simulink model "adrc_plant"  (R2026a)
settings: Solver=FixedStepDiscrete  StartTime=0  StopTime=6  FixedStep=0.004
settings Model: Creator=Aethor_ca  LastModifiedBy=Aethor_ca
settings DebuggingCC: AlgebraicLoopMsg=error
settings ModelReferenceCC: ModelReferenceMinAlgLoopOccurrences=on
settings GRTTargetCC: CombineOutputUpdateFcns=off

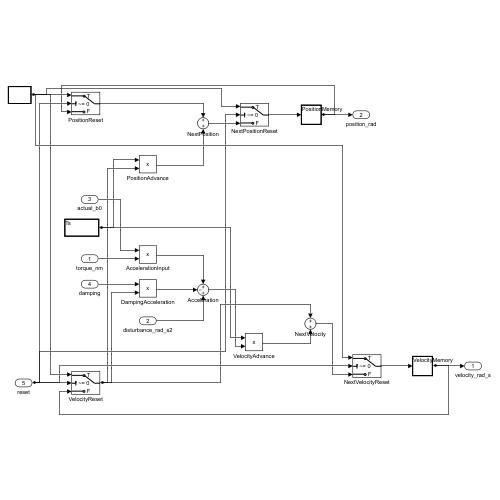
[thumbnail: Simulink's stored preview of the top-level diagram]
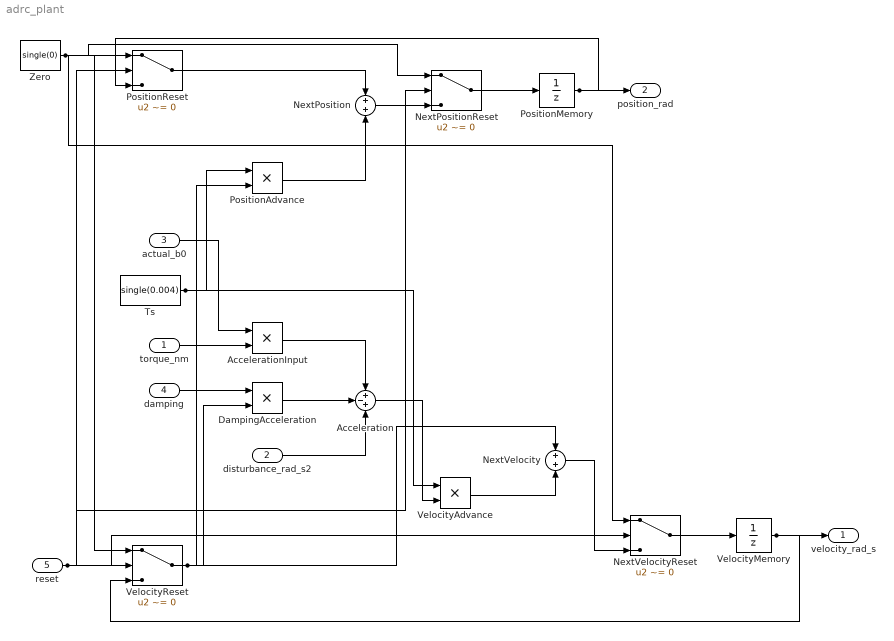
== system adrc_plant ==
  torque_nm : Inport  OutDataTypeStr=single  PortDimensions=1  SampleTime=0.004
  disturbance_rad_s2 : Inport  Port=2  OutDataTypeStr=single  PortDimensions=1  SampleTime=0.004
  actual_b0 : Inport  Port=3  OutDataTypeStr=single  PortDimensions=1  SampleTime=0.004
  damping : Inport  Port=4  OutDataTypeStr=single  PortDimensions=1  SampleTime=0.004
  reset : Inport  Port=5  OutDataTypeStr=uint8  PortDimensions=1  SampleTime=0.004
  Acceleration : Sum  Inputs=+-+  OutDataTypeStr=single
  AccelerationInput : Product  Inputs=**  OutDataTypeStr=single
  DampingAcceleration : Product  Inputs=**  OutDataTypeStr=single
  NextPosition : Sum  OutDataTypeStr=single
  NextPositionReset : Switch  Criteria=u2 ~= 0  OutDataTypeStr=single  SaturateOnIntegerOverflow=off  InputSameDT=off
  NextVelocity : Sum  OutDataTypeStr=single
  NextVelocityReset : Switch  Criteria=u2 ~= 0  OutDataTypeStr=single  SaturateOnIntegerOverflow=off  InputSameDT=off
  PositionAdvance : Product  Inputs=**  OutDataTypeStr=single
  PositionMemory : UnitDelay  InitialCondition=single(0)  SampleTime=0.004
  PositionReset : Switch  Criteria=u2 ~= 0  OutDataTypeStr=single  SaturateOnIntegerOverflow=off  InputSameDT=off
  Ts : Constant  Value=single(0.004)  OutDataTypeStr=single
  VelocityAdvance : Product  Inputs=**  OutDataTypeStr=single
  VelocityMemory : UnitDelay  InitialCondition=single(0)  SampleTime=0.004
  VelocityReset : Switch  Criteria=u2 ~= 0  OutDataTypeStr=single  SaturateOnIntegerOverflow=off  InputSameDT=off
  Zero : Constant  Value=single(0)  OutDataTypeStr=single
  velocity_rad_s : Outport  OutDataTypeStr=single
  position_rad : Outport  Port=2  OutDataTypeStr=single
  wires:
  Acceleration/1 -> VelocityAdvance/2
  actual_b0/1 -> AccelerationInput/1
  VelocityAdvance/1 -> NextVelocity/2
  Zero/1 -> NextVelocityReset/1, NextPositionReset/1, VelocityReset/1, PositionReset/1
  torque_nm/1 -> AccelerationInput/2
  AccelerationInput/1 -> Acceleration/1
  reset/1 -> NextVelocityReset/2, NextPositionReset/2, VelocityReset/2, PositionReset/2
  PositionReset/1 -> NextPosition/1
  VelocityReset/1 -> NextVelocity/1, DampingAcceleration/2, PositionAdvance/2
  NextVelocity/1 -> NextVelocityReset/3
  Ts/1 -> VelocityAdvance/1, PositionAdvance/1
  damping/1 -> DampingAcceleration/1
  PositionAdvance/1 -> NextPosition/2
  DampingAcceleration/1 -> Acceleration/2
  disturbance_rad_s2/1 -> Acceleration/3
  NextPosition/1 -> NextPositionReset/3
  NextPositionReset/1 -> PositionMemory/1
  PositionMemory/1 -> PositionReset/3, position_rad/1
  NextVelocityReset/1 -> VelocityMemory/1
  VelocityMemory/1 -> VelocityReset/3, velocity_rad_s/1
